simulink model "MMC_200Cell_WB_Par_Ccode"  (R2024b)
settings: Solver=FixedStepAuto  StartTime=0.0  StopTime=5  FixedStep=Ts  RelTol=1e-3
PostLoadFcn:
  | init_MMC_HVDC_200; load MMC_busStructures.mat;
InitFcn:
  | init_MMC_HVDC_200; load MMC_busStructures.mat;
values from neighbouring files (symbols this model uses):
  Ts = 35e-6    (= 3.5e-05)    [init_MMC_HVDC_200.m]
libraries: simetranss x1
Description:
  | MMC model
settings Model: ARTEMISmethode_block_infos=$$__separator__$$  ExplicitPartitioning=on  Creator=Kyle  LastModifiedBy=CD8435
settings SolverCC: ConcurrentTasks=on  AlgebraicLoopSolver=TrustRegion
settings DataIOCC: LimitDataPoints=on  SaveFormat=Array  SignalLoggingSaveFormat=ModelDataLogs  SaveOutput=off  SignalLogging=off  DSMLogging=off  SaveTime=off  ReturnWorkspaceOutputs=off
settings OptimizationCC: BlockReduction=off  OptimizeBlockIOStorage=off  BufferReuse=off  GlobalBufferReuse=off  ExpressionFolding=off  ExpressionDepthLimit=2147483647  LocalBlockOutputs=off  ZeroExternalMemoryAtStartup=off  ZeroInternalMemoryAtStartup=off  LifeSpan=inf  OptimizeDataStoreBuffers=off  BusAssignmentInplaceUpdate=off
settings DebuggingCC: UnderspecifiedInitializationDetection=Classic  MergeDetectMultiDrivingBlocksExec=none  FcnCallInpInsideContextMsg=warning  UnconnectedInputMsg=warning  UnconnectedOutputMsg=warning  UnconnectedLineMsg=warning  StateNameClashWarn=warning  SFUnexpectedBacktrackingDiag=warning  SFNoUnconditionalDefaultTransitionDiag=warning  SFExecutionAtInitializationDiag=none  ArithmeticOperatorsInVariantConditions=warning
settings HardwareCC: ProdBitPerPointer=32  ProdBitPerSizeT=32  ProdBitPerPtrDiffT=32  ProdLargestAtomicFloat=None  ProdIntDivRoundTo=Undefined  ProdEndianess=Unspecified  ProdWordSize=32  ProdHWDeviceType=32-bit Generic
settings ModelReferenceCC: EnableRefExpFcnMdlSchedulingChecks=on  PropagateSignalLabelsOutOfModel=off
settings SFSimCC: SimUseLocalCustomCode=off  CustomCodeUndefinedFunction=UseInterfaceOnly
settings RTWCC: ProfileTLC=on  TLCCoverage=on  TLCAssert=on  RTWUseLocalCustomCode=off  TargetLang=C++  GPUComputeCapability=3.5
settings CodeAppCC: StateflowObjectComments=on
settings GRTTargetCC: TargetLangStandard=C++11 (ISO)  MatFileLogging=off  CodeInterfacePackaging=C++ class
settings ConfigComp: CovMetricSettings=dw  CovSaveCumulativeToWorkspaceVar=on  CovSaveSingleToWorkspaceVar=on  CovExternalEMLEnable=off
settings SimscapeCC: SimscapeNormalizeSystem=off

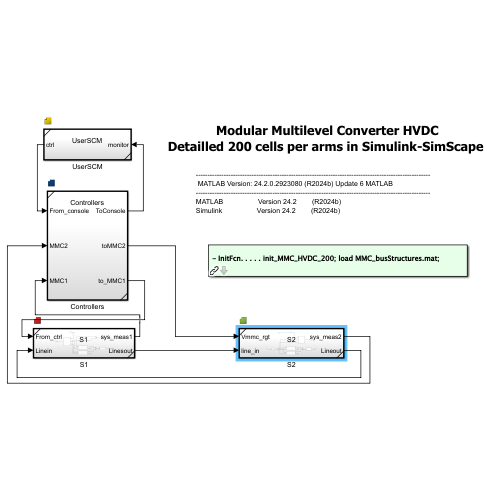
[thumbnail: Simulink's stored preview of the top-level diagram]
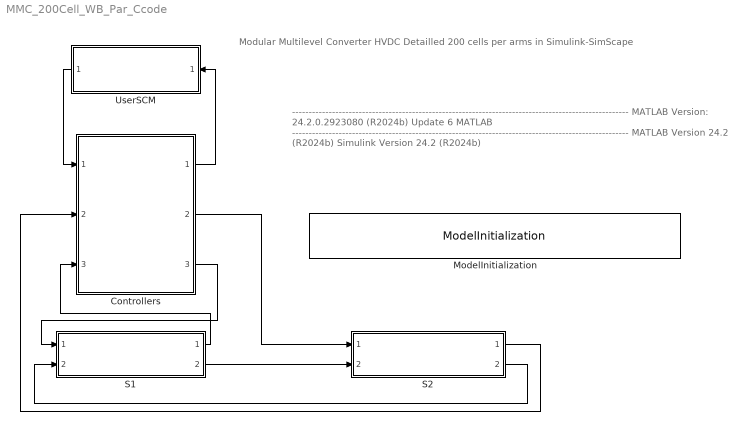
== system MMC_200Cell_WB_Par_Ccode ==
  note: -----------------------------------------------------------------------------------------------------
      |  MATLAB Version: 24.2.0.2923080 (R2024b) Update 6 MATLAB   -----------------------------------------------------------------------------------------------------
      | MATLAB                  Version 24.2        (R2024b)
      | Simulink                  Version 24.2        (R2024b)
  note: Modular Multilevel Converter HVDC
      |  Detailled 200 cells per arms in Simulink-SimScape
  Controllers : Subsystem  TreatAsAtomicUnit=on  SystemSampleTime=Ts  ReferencedSubsystem=Controllers
  ModelInitialization : simetranss/Usefulls/ModelInitialization  InitFcnX=init_MMC_HVDC_200; load MMC_busStructures.mat;  prel=off  posl=on  inif=on  strf=off
  S1 : Subsystem  TreatAsAtomicUnit=on  SystemSampleTime=Ts  ReferencedSubsystem=S1
  S2 : Subsystem  TreatAsAtomicUnit=on  SystemSampleTime=Ts  ReferencedSubsystem=S2
  UserSCM : Subsystem  TreatAsAtomicUnit=on  SystemSampleTime=Ts  ReferencedSubsystem=UserSCM
  wires:
  UserSCM/1 -> Controllers/1
  Controllers/1 -> UserSCM/1
  Controllers/3 -> S1/1
  S1/1 -> Controllers/3
  Controllers/2 -> S2/1
  S2/1 -> Controllers/2
  S2/2 -> S1/2
  S1/2 -> S2/2
